simulink model "quad_model"  (Simulink 7.8)
settings: Solver=ode45  StartTime=0.0  StopTime=10.0  RelTol=1e-3
values from neighbouring files (symbols this model uses):
  Ts = 0.02    [kostas_malakies.mat]    (also in kostas_malakies2.mat; main.m; main_last.m; matlab.mat = 0.08)
libraries: Hqaud_model_LIB_SI x1
settings Model: Creator=burrimi  LastModifiedBy=burrimi

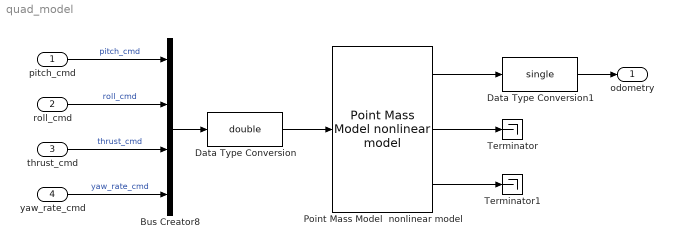
== system quad_model ==
  pitch_cmd : Inport  OutDataTypeStr=single  PortDimensions=1  SampleTime=Ts
  roll_cmd : Inport  Port=2  OutDataTypeStr=single  PortDimensions=1  SampleTime=Ts
  thrust_cmd : Inport  Port=3  OutDataTypeStr=single  PortDimensions=1  SampleTime=Ts
  yaw_rate_cmd : Inport  Port=4  OutDataTypeStr=single  PortDimensions=1  SampleTime=Ts
  Bus Creator8 : BusCreator
  Data Type Conversion : DataTypeConversion  OutDataTypeStr=double
  Data Type Conversion1 : DataTypeConversion  OutDataTypeStr=single
  Point Mass Model  nonlinear model : Hqaud_model_LIB_SI/Point Mass Model  nonlinear model
  Terminator : Terminator
  Terminator1 : Terminator
  odometry : Outport  OutDataTypeStr=single  SampleTime=Ts
  wires:
  pitch_cmd/1 -> Bus Creator8/1  "pitch_cmd"
  roll_cmd/1 -> Bus Creator8/2  "roll_cmd"
  thrust_cmd/1 -> Bus Creator8/3  "thrust_cmd"
  yaw_rate_cmd/1 -> Bus Creator8/4  "yaw_rate_cmd"
  Bus Creator8/1 -> Data Type Conversion/1
  Data Type Conversion1/1 -> odometry/1
  Data Type Conversion/1 -> Point Mass Model  nonlinear model/1
  Point Mass Model  nonlinear model/1 -> Data Type Conversion1/1
  Point Mass Model  nonlinear model/3 -> Terminator1/1
  Point Mass Model  nonlinear model/2 -> Terminator/1
